simulink model "sampleModel1986"  (R2022a)
settings: Solver=FixedStepAuto  StartTime=0.0  StopTime=10.0  RelTol=1e-3
undefined symbols (not defined in the file): DiscIntNeverNeededParam, magnitude, Newton, Raphson
libraries: simulink x65, slpidlib x29
(part 1 of 4)
settings Model: SimulationMode=software-in-the-loop (sil)  Creator=lenovo  LastModifiedBy=TSMC
settings DataIOCC: InspectSignalLogs=on  SignalLoggingName=logsOut
settings OptimizationCC: DefaultParameterBehavior=Inlined  EnhancedBackFolding=on  PassReuseOutputArgsAs=Individual arguments  ZeroExternalMemoryAtStartup=off  ZeroInternalMemoryAtStartup=off  OptimizeBlockOrder=speed  DifferentSizesBufferReuse=on  OptimizationCustomize=off  EfficientTunableParamExpr=on
settings DebuggingCC: ParameterTunabilityLossMsg=error  UnconnectedInputMsg=warning  UnconnectedOutputMsg=warning  UnconnectedLineMsg=warning
settings ModelReferenceCC: UpdateModelReferenceTargets=Force
settings SFSimCC: MATLABDynamicMemAlloc=off
settings RTWCC: SystemTargetFile=ert.tlc  TemplateMakefile=ert_default_tmf  GenerateReport=on  IncludeHyperlinkInReport=on  GenerateTraceInfo=on  DLArmComputeVersion=19.05
settings CodeAppCC: ForceParamTrailComments=on  IgnoreCustomStorageClasses=off  OperatorAnnotations=on  SimulinkDataObjDesc=on  SFDataObjDesc=on  InsertBlockDesc=on
settings ERTTargetCC: TargetLangStandard=C99 (ISO)  GenerateSampleERTMain=on  SupportContinuousTime=on  InlinedParameterPlacement=NonHierarchical  ERTCustomFileTemplate=example_file_process.tlc

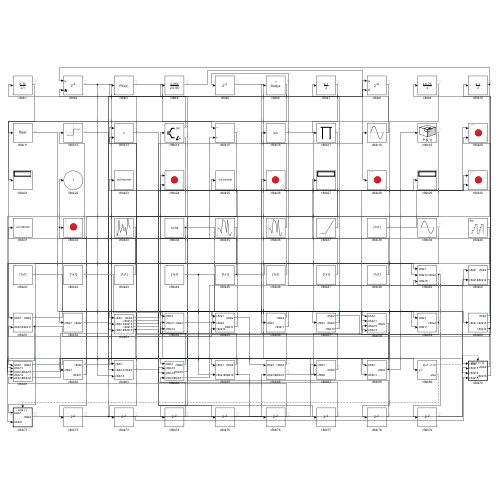
[thumbnail: Simulink's stored preview of the top-level diagram]
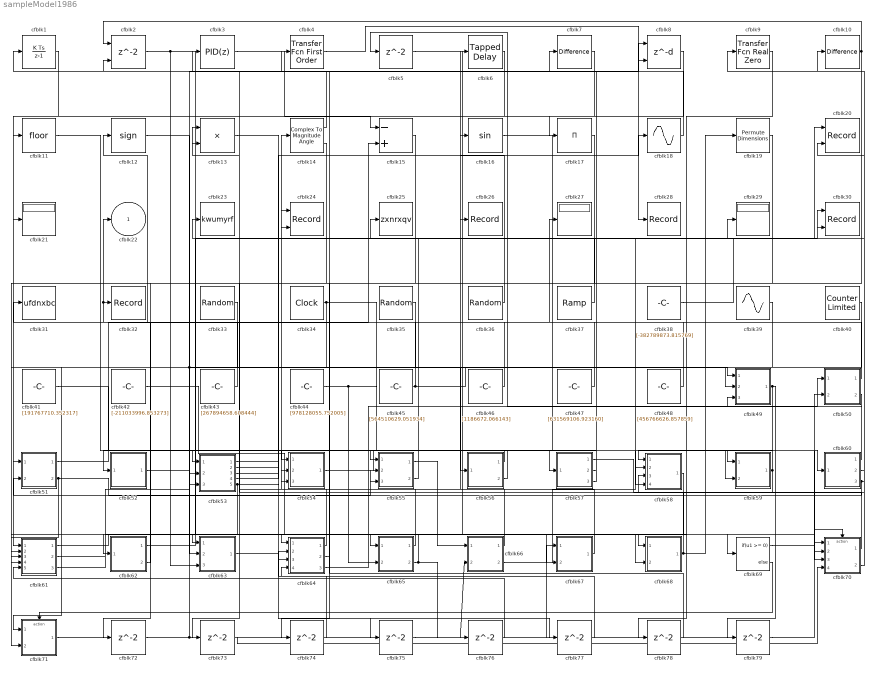
== system sampleModel1986 ==
  cfblk1 : DiscreteIntegrator  ICPrevOutput=DiscIntNeverNeededParam  ICPrevScaledInput=DiscIntNeverNeededParam
  cfblk10 : simulink/Discrete/Difference  ICPrevInput=0.0  OutMin=[]  OutMax=[]  OutDataTypeStr=Inherit: Inherit via back propagation  OutDataType=fixdt(1, 16)  OutScaling=2^-10  DoSatur=off
  cfblk11 : Rounding
  cfblk12 : Signum
  cfblk13 : Product  Inputs=**
  cfblk14 : ComplexToMagnitudeAngle
  cfblk15 : Sum  Inputs=-+
  cfblk16 : Trigonometry
  cfblk17 : Product  Inputs=*
  cfblk18 : Sin  TimeSource=Use external signal  SampleTime=0
  cfblk19 : PermuteDimensions
  cfblk2 : Delay  ShowEnablePort=on  SampleTime=1
      settings: InputPortMap=u0,e6
  cfblk20 : Record  FileSettingsInternal="{\"entries\":[{\"content\":{\"excelSettings\":{\"content\":{},\"type\":\"Streamout.ExcelSettings\"}},\"type\":\"Streamout.FileSettingStorage\",\"uuid\":\"1dca6e3d-3929-4a9b-a58f-98e31c8e366e\"}],\"packageUris\":[\"http://schema.mathworks.com/mf0/streamout_blocks/R2020a\"],\"version\":\"1.0\"}"  Layout=[1 1]  SignalsInternal="{\"entries\":[{\"content\":{\"signals\":[]},\"type\":\"RecordBlkView.InputSignals\",\"uuid\":\"f96b82a6-c829-4707-99bd-2f6ef44443c5\"}],\"packageUris\":[\"http://schema.mathworks.com/mf0/streamout_blocks/R2020a\"],\"version\":\"1.0\"}"  VisualizationBindings="{\"xyplotplugin\":{\"info\":[{\"series\":[],\"subplotID\":1}]}}"  CompatibilityTag=XY  st=-1
  cfblk21 : Display
  cfblk23 : ToWorkspace  VariableName=kwumyrf  SaveFormat=Timeseries  SampleTime=-1
  cfblk24 : Record  FileSettingsInternal="{\"entries\":[{\"content\":{\"excelSettings\":{\"content\":{},\"type\":\"Streamout.ExcelSettings\"}},\"type\":\"Streamout.FileSettingStorage\",\"uuid\":\"2952f6c9-f0ad-4b3b-947f-ff8e5daf63b8\"}],\"packageUris\":[\"http://schema.mathworks.com/mf0/streamout_blocks/R2020a\"],\"version\":\"1.0\"}"  Layout=[1 1]  SignalsInternal="{\"entries\":[{\"content\":{\"signals\":[]},\"type\":\"RecordBlkView.InputSignals\",\"uuid\":\"72db522a-7474-45f0-8336-b7d99dcf0ae2\"}],\"packageUris\":[\"http://schema.mathworks.com/mf0/streamout_blocks/R2020a\"],\"version\":\"1.0\"}"  VisualizationBindings="{\"xyplotplugin\":{\"info\":[{\"series\":[],\"subplotID\":1}]}}"  CompatibilityTag=XY  st=-1
  cfblk25 : ToWorkspace  VariableName=zxnrxqv  SaveFormat=Timeseries  SampleTime=-1
  cfblk26 : Record  FileSettingsInternal="{\"entries\":[{\"content\":{\"excelSettings\":{\"content\":{},\"type\":\"Streamout.ExcelSettings\"}},\"type\":\"Streamout.FileSettingStorage\",\"uuid\":\"125c1273-ce01-40e0-820a-1ab6df99f7c8\"}],\"packageUris\":[\"http://schema.mathworks.com/mf0/streamout_blocks/R2020a\"],\"version\":\"1.0\"}"  SignalsInternal="{\"entries\":[{\"content\":{\"signals\":[]},\"type\":\"RecordBlkView.InputSignals\",\"uuid\":\"39647610-03c1-4d8e-aa54-680a15d5938d\"}],\"packageUris\":[\"http://schema.mathworks.com/mf0/streamout_blocks/R2020a\"],\"version\":\"1.0\"}"  VisualizationBindings="{\"sparklinesplugin\":{\"info\":[{\"bindingParametersList\":[],\"subplotID\":1}]}}"
  cfblk27 : Display
  cfblk28 : Record  FileSettingsInternal="{\"entries\":[{\"content\":{\"excelSettings\":{\"content\":{},\"type\":\"Streamout.ExcelSettings\"}},\"type\":\"Streamout.FileSettingStorage\",\"uuid\":\"d5079e4d-954f-4e3f-aebb-353b75416782\"}],\"packageUris\":[\"http://schema.mathworks.com/mf0/streamout_blocks/R2020a\"],\"version\":\"1.0\"}"  SignalsInternal="{\"entries\":[{\"content\":{\"signals\":[]},\"type\":\"RecordBlkView.InputSignals\",\"uuid\":\"3476c6fd-dd80-4faf-a5c2-c4212778116c\"}],\"packageUris\":[\"http://schema.mathworks.com/mf0/streamout_blocks/R2020a\"],\"version\":\"1.0\"}"  VisualizationBindings="{\"sparklinesplugin\":{\"info\":[{\"bindingParametersList\":[],\"subplotID\":1}]}}"
  cfblk29 : Display
  cfblk3 : slpidlib/PID Controller  Controller=PID  Form=Parallel  TimeDomain=Discrete-time  UseExternalTs=off  SampleTime=1  IntegratorMethod=Forward Euler  FilterMethod=Forward Euler  ControllerParametersSource=internal  P=1  I=1  UseKiTs=off  D=0  N=100  UseFilter=on  TunerSelectOption=Transfer Function Based (PID Tuner App)  InitialConditionSource=internal  InitialConditionForIntegrator=0  InitialConditionForFilter=0  DifferentiatorICPrevScaledInput=0  ExternalReset=none  TrackingMode=off  Kt=1  LimitOutput=off  SatLimitsSource=internal  UpperSaturationLimit=inf  LowerSaturationLimit=-inf  LinearizeAsGain=off  AntiWindupMode=none  Kb=1  POutMin=[]  POutMax=[]  IOutMin=[]  IOutMax=[]  DOutMin=[]  DOutMax=[]  NOutMin=[]  NOutMax=[]  SumOutMin=[]  SumOutMax=[]  SaturationOutMin=[]  SaturationOutMax=[]  PParamMin=[]  PParamMax=[]  IParamMin=[]  IParamMax=[]  DParamMin=[]  DParamMax=[]  NParamMin=[]  NParamMax=[]  KbParamMin=[]  KbParamMax=[]  KtParamMin=[]  KtParamMax=[]  KbOutMin=[]  KbOutMax=[]  KtOutMin=[]  KtOutMax=[]  IntegratorOutMin=[]  IntegratorOutMax=[]  FilterOutMin=[]  FilterOutMax=[]  SumI1OutMin=[]  SumI1OutMax=[]  SumI2OutMin=[]  SumI2OutMax=[]  SumI3OutMin=[]  SumI3OutMax=[]  SumI4OutMin=[]  SumI4OutMax=[]  SumDOutMin=[]  SumDOutMax=[]  DifferentiatorOutMin=[]  DifferentiatorOutMax=[]  FilterDiffOutCoefMin=[]  FilterDiffOutCoefMax=[]  ReciprocalOutMin=[]  ReciprocalOutMax=[]  SumDenOutMin=[]  SumDenOutMax=[]  SumNumOutMin=[]  SumNumOutMax=[]  DivideOutMin=[]  DivideOutMax=[]  UdiffTsProdOutMin=[]  UdiffTsProdOutMax=[]  NTsProdOutMin=[]  NTsProdOutMax=[]  UintegralTsProdOutMin=[]  UintegralTsProdOutMax=[]  UngainTsProdOutMin=[]  UngainTsProdOutMax=[]  IntegratorContinuousStateAttributes=''  IntegratorStateMustResolveToSignalObject=off  IntegratorRTWStateStorageClass=Auto  FilterContinuousStateAttributes=''  FilterStateMustResolveToSignalObject=off  FilterRTWStateStorageClass=Auto  ParallelPVariant=InternalParameters  IdealPVariant=Disabled  IVariant=InternalParameters  DVariant=InternalParameters  IntegratorVariant=Discrete  SatVariant=Disabled  AWVariant=Passthrough  PCopyVariant=Disabled  TRVariant=Disabled  FdbkBlocksVariant=Forward  IdealPFdbkVariant=Disabled  SatFdbkVariant=Disabled  DerivativeFilterVariant=ForwardEulerFilter  NVariant=InternalParameters  NCopyVariant=Disabled  FilterICVariant=InternalICsFilter  IntegratorICVariant=InternalICs  ExternalResetVariant=Disabled  TRSumVariant=Passthrough  SumFdbkVariant=Disabled  SumVariant=Sum_PID  TsampFilterVariant=InternalTs  TsampNgainVariant=Passthrough  TsampIntegralVariant=Passthrough  ExternalSaturationOutDataTypeStr=Inherit: Same as second input  aMode=0
  cfblk30 : Record  FileSettingsInternal="{\"entries\":[{\"content\":{\"excelSettings\":{\"content\":{},\"type\":\"Streamout.ExcelSettings\"}},\"type\":\"Streamout.FileSettingStorage\",\"uuid\":\"e2760d90-3872-4efb-b71f-af873bcd0c0f\"}],\"packageUris\":[\"http://schema.mathworks.com/mf0/streamout_blocks/R2020a\"],\"version\":\"1.0\"}"  Layout=[1 1]  SignalsInternal="{\"entries\":[{\"content\":{\"signals\":[]},\"type\":\"RecordBlkView.InputSignals\",\"uuid\":\"4f91cc43-4657-47a6-9057-0df5bd7a9694\"}],\"packageUris\":[\"http://schema.mathworks.com/mf0/streamout_blocks/R2020a\"],\"version\":\"1.0\"}"  VisualizationBindings="{\"xyplotplugin\":{\"info\":[{\"series\":[],\"subplotID\":1}]}}"  CompatibilityTag=XY  st=-1
  cfblk31 : ToWorkspace  VariableName=ufdnxbc  SaveFormat=Timeseries  SampleTime=-1
  cfblk32 : Record  FileSettingsInternal="{\"entries\":[{\"content\":{\"excelSettings\":{\"content\":{},\"type\":\"Streamout.ExcelSettings\"}},\"type\":\"Streamout.FileSettingStorage\",\"uuid\":\"319a848f-b9c4-4916-ac33-385dec724fbf\"}],\"packageUris\":[\"http://schema.mathworks.com/mf0/streamout_blocks/R2020a\"],\"version\":\"1.0\"}"  SignalsInternal="{\"entries\":[{\"content\":{\"signals\":[]},\"type\":\"RecordBlkView.InputSignals\",\"uuid\":\"3da1b3d0-60d1-46be-bad3-5ce6aab02480\"}],\"packageUris\":[\"http://schema.mathworks.com/mf0/streamout_blocks/R2020a\"],\"version\":\"1.0\"}"  VisualizationBindings="{\"sparklinesplugin\":{\"info\":[{\"bindingParametersList\":[],\"subplotID\":1}]}}"
  cfblk33 : UniformRandomNumber  Minimum=[-1660380243.900626]  Maximum=[7164102365.047249]  Seed=[69049731.000000]  SampleTime=0.1
  cfblk34 : DigitalClock
  cfblk35 : RandomNumber  Mean=[-39556.035866]  Variance=[56886.779611]  Seed=[852067175.000000]  SampleTime=0.1
  cfblk36 : RandomNumber  Mean=[-57488.389087]  Variance=[56185.308516]  Seed=[940335256.000000]  SampleTime=0.1
  cfblk37 : simulink/Sources/Ramp  slope=[8074.641481]  start=[17.613645]  InitialOutput=[-350516.986257]
  cfblk38 : Constant  Value=[-382789873.815769]  SampleTime=1
  cfblk39 : Sin  Amplitude=[560591672.625923]  Bias=[-94874390.999346]  SampleTime=0
  cfblk4 : simulink/Discrete/Transfer Fcn First Order  PoleZ=0.95  ICPrevOutput=0.0  DoSatur=off
  cfblk40 : simulink/Sources/Counter Limited  uplimit=[971.000000]  tsamp=-1
  cfblk41 : Constant  Value=[191767710.352317]  SampleTime=1
  cfblk42 : Constant  Value=[-211033996.853273]  SampleTime=1
  cfblk43 : Constant  Value=[267894658.608444]  SampleTime=1
  cfblk44 : Constant  Value=[978128055.752005]  SampleTime=1
  cfblk45 : Constant  Value=[564510629.051934]  SampleTime=1
  cfblk46 : Constant  Value=[1186672.066143]  SampleTime=1
  cfblk47 : Constant  Value=[631569106.923160]  SampleTime=1
  cfblk48 : Constant  Value=[456766626.857859]  SampleTime=1
  cfblk49 : Subsystem
  cfblk{5,72..79} (9 alike) : Delay  SampleTime=1
  cfblk50 : Subsystem
  cfblk51 : Subsystem
  cfblk52 : Subsystem
  cfblk53 : Subsystem
  cfblk54 : Subsystem
  cfblk55 : Subsystem
  cfblk56 : Subsystem
  cfblk57 : Subsystem
  cfblk58 : Subsystem
  cfblk59 : Subsystem
  cfblk6 : simulink/Discrete/Tapped Delay  vinit=0.0  samptime=-1  NumDelays=1  DelayOrder=Oldest  includeCurrent=off
  cfblk60 : Subsystem
  cfblk61 : Subsystem
  cfblk62 : Subsystem
  cfblk63 : Subsystem
  cfblk64 : Subsystem
  cfblk65 : Subsystem
  cfblk66 : Subsystem
  cfblk67 : Subsystem
  cfblk68 : Subsystem
  cfblk69 : If  IfExpression=u1 >= 0  SampleTime=1
  cfblk7 : simulink/Discrete/Difference  ICPrevInput=0.0  OutMin=[]  OutMax=[]  OutDataTypeStr=Inherit: Inherit via back propagation  OutDataType=fixdt(1, 16)  OutScaling=2^-10  DoSatur=off
  cfblk70 : Subsystem  TreatAsAtomicUnit=on
  cfblk71 : Subsystem  TreatAsAtomicUnit=on
  cfblk8 : Delay  DelayLengthSource=Input port  SampleTime=1
      settings: InputPortMap=u0,p1
  cfblk9 : simulink/Discrete/Transfer Fcn Real Zero  ZeroZ=0.75  ICPrevInput=0.0  DoSatur=off
      settings: SourceProductBaseCode=SL
  cfblk22 : Outport
  wires:
  cfblk43/1 -> cfblk22/1, cfblk32/1
  cfblk55/1(cfblk2) -> cfblk66/1(cfblk1)
  cfblk6/1 -> cfblk61/1(cfblk1)
  cfblk59/1(cfblk2) -> cfblk58/1(cfblk1), cfblk55/3(cfblk10)
  cfblk60/1(cfblk2) -> cfblk5/1
  cfblk57/1(cfblk2) -> cfblk10/1
  cfblk16/1 -> cfblk58/2(cfblk11)
  cfblk4/1 -> cfblk28/1
  cfblk9/1 -> cfblk68/1(cfblk1)
  cfblk5/1 -> cfblk69/1
  cfblk2/1 -> cfblk64/1(cfblk1), cfblk63/3(cfblk13)
  cfblk18/1 -> cfblk7/1
  cfblk71/1(cfblk2) -> cfblk66/2(cfblk15), cfblk53/2(cfblk11)
  cfblk56/1(cfblk2) -> cfblk52/1(cfblk1)
  cfblk54/1(cfblk2) -> cfblk60/1(cfblk1)
  cfblk60/2(cfblk13) -> cfblk9/1
  cfblk44/1 -> cfblk70/1(cfblk1), cfblk65/2(cfblk15)
  cfblk68/1(cfblk2) -> cfblk13/1, cfblk19/1
  cfblk67/1(cfblk2) -> cfblk6/1
  cfblk61/1(cfblk2) -> cfblk68/2(cfblk11)
  cfblk41/1 -> cfblk57/1(cfblk1)
  cfblk65/1(cfblk2) -> cfblk13/2
  cfblk40/1 -> cfblk56/1(cfblk1)
  cfblk42/1 -> cfblk70/3(cfblk14)
  cfblk8/1 -> cfblk17/1
  cfblk62/1(cfblk2) -> cfblk30/1
  cfblk33/1 -> cfblk71/1(cfblk1), cfblk53/3(cfblk12)
  cfblk3/1 -> cfblk15/1
  cfblk14/1 -> cfblk1/1
  cfblk1/1 -> cfblk21/1
  cfblk60/3(cfblk14) -> cfblk25/1, cfblk51/2(cfblk10)
  cfblk62/2(cfblk11) -> cfblk31/1
  cfblk7/1 -> cfblk11/1
  cfblk45/1 -> cfblk49/1(cfblk1), cfblk3/1
  cfblk61/2(cfblk15) -> cfblk65/1(cfblk1)
  cfblk35/1 -> cfblk64/3(cfblk14)
  cfblk12/1 -> cfblk49/2(cfblk14)
  cfblk56/2(cfblk11) -> cfblk53/1(cfblk1)
  cfblk39/1 -> cfblk61/2(cfblk11)
  cfblk50/1(cfblk2) -> cfblk27/1
  cfblk38/1 -> cfblk20/1
  cfblk10/1 -> cfblk2/1, cfblk62/1(cfblk1)
  cfblk70/1(cfblk2) -> cfblk58/3(cfblk12)
  cfblk66/1(cfblk2) -> cfblk14/1
  cfblk49/1(cfblk2) -> cfblk78/1, cfblk79/1
  cfblk46/1 -> cfblk24/1
  cfblk50/2(cfblk14) -> cfblk49/3(cfblk15)
  cfblk15/1 -> cfblk71/2(cfblk8)
  cfblk47/1 -> cfblk12/1
  cfblk36/1 -> cfblk16/1
  cfblk57/2(cfblk9) -> cfblk54/1(cfblk1)
  cfblk65/2(cfblk16) -> cfblk63/1(cfblk1), cfblk76/1
  cfblk70/2(cfblk16) -> cfblk20/2
  cfblk13/1 -> cfblk55/1(cfblk1)
  cfblk66/2(cfblk16) -> cfblk30/2
  cfblk48/1 -> cfblk26/1
  cfblk17/1 -> cfblk63/2(cfblk12)
  cfblk64/1(cfblk2) -> cfblk54/2(cfblk11)
  cfblk57/3(cfblk10) -> cfblk4/1
  cfblk61/3(cfblk16) -> cfblk8/1
  cfblk52/1(cfblk2) -> cfblk8/2
  cfblk64/2(cfblk16) -> cfblk54/3(cfblk12)
  cfblk11/1 -> cfblk58/4(cfblk13)
  cfblk53/1(cfblk2) -> cfblk59/1(cfblk1)
  cfblk51/1(cfblk2) -> cfblk15/2
  cfblk37/1 -> cfblk23/1
  cfblk64/3(cfblk17) -> cfblk50/1(cfblk1)
  cfblk51/2(cfblk11) -> cfblk61/3(cfblk12), cfblk55/2(cfblk9)
  cfblk53/2(cfblk13) -> cfblk67/2(cfblk8)
  cfblk53/3(cfblk14) -> cfblk18/1
  cfblk34/1 -> cfblk51/1(cfblk1), cfblk59/2(cfblk11)
  cfblk55/2(cfblk11) -> cfblk24/2
  cfblk53/4(cfblk15) -> cfblk29/1
  cfblk53/5(cfblk16) -> cfblk61/4(cfblk13), cfblk77/1
  cfblk69/1 -> cfblk70/Action
  cfblk69/2 -> cfblk71/Action
  cfblk58/1(cfblk2) -> cfblk72/1
  cfblk72/1 -> cfblk70/2(cfblk13)
  cfblk14/2 -> cfblk73/1
  cfblk73/1 -> cfblk70/4(cfblk15)
  cfblk19/1 -> cfblk74/1
  cfblk74/1 -> cfblk64/2(cfblk13)
  cfblk63/1(cfblk2) -> cfblk75/1
  cfblk75/1 -> cfblk67/1(cfblk1)
  cfblk76/1 -> cfblk61/5(cfblk14)
  cfblk77/1 -> cfblk64/4(cfblk15)
  cfblk78/1 -> cfblk2/2
  cfblk79/1 -> cfblk50/2(cfblk13)

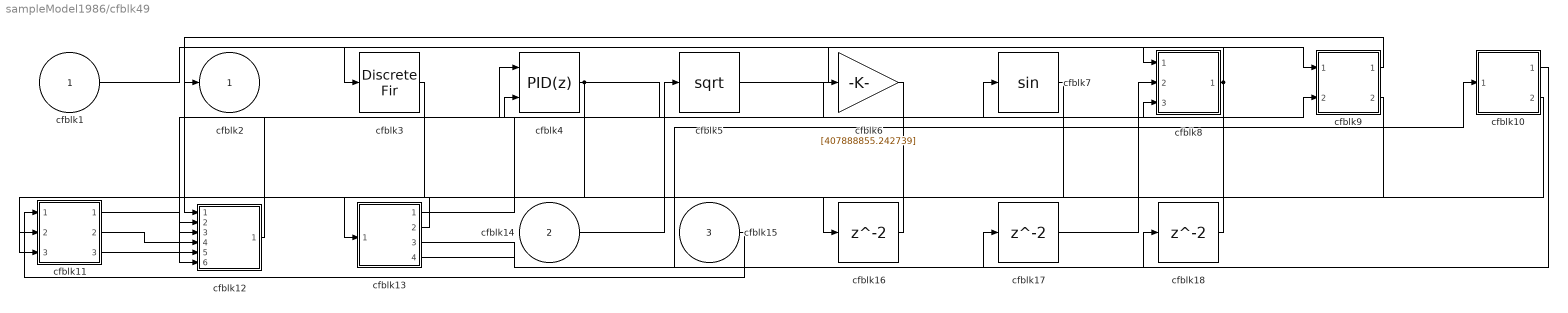
== system sampleModel1986/cfblk49 ==
  cfblk1 : Inport
  cfblk14 : Inport  Port=2
  cfblk15 : Inport  Port=3
  cfblk10 : Subsystem
  cfblk11 : Subsystem
  cfblk12 : Subsystem
  cfblk13 : Subsystem
  cfblk16 : Delay  SampleTime=1
  cfblk17 : Delay  SampleTime=1
  cfblk18 : Delay  SampleTime=1
  cfblk3 : DiscreteFir  SampleTime=1
  cfblk4 : slpidlib/PID Controller (2DOF)  Controller=PID  Form=Parallel  TimeDomain=Discrete-time  UseExternalTs=off  SampleTime=1  IntegratorMethod=Forward Euler  FilterMethod=Forward Euler  ControllerParametersSource=internal  P=1  I=1  UseKiTs=off  D=0  N=100  UseFilter=on  b=1  c=1  TunerSelectOption=Transfer Function Based (PID Tuner App)  InitialConditionSource=internal  InitialConditionForIntegrator=0  InitialConditionForFilter=0  DifferentiatorICPrevScaledInput=0  ExternalReset=none  TrackingMode=off  Kt=1  LimitOutput=off  SatLimitsSource=internal  UpperSaturationLimit=inf  LowerSaturationLimit=-inf  LinearizeAsGain=off  AntiWindupMode=none  Kb=1  POutMin=[]  POutMax=[]  IOutMin=[]  IOutMax=[]  DOutMin=[]  DOutMax=[]  NOutMin=[]  NOutMax=[]  bOutMin=[]  bOutMax=[]  cOutMin=[]  cOutMax=[]  SumOutMin=[]  SumOutMax=[]  SaturationOutMin=[]  SaturationOutMax=[]  PParamMin=[]  PParamMax=[]  IParamMin=[]  IParamMax=[]  DParamMin=[]  DParamMax=[]  NParamMin=[]  NParamMax=[]  bParamMin=[]  bParamMax=[]  cParamMin=[]  cParamMax=[]  KbParamMin=[]  KbParamMax=[]  KtParamMin=[]  KtParamMax=[]  KbOutMin=[]  KbOutMax=[]  KtOutMin=[]  KtOutMax=[]  IntegratorOutMin=[]  IntegratorOutMax=[]  FilterOutMin=[]  FilterOutMax=[]  SumI1OutMin=[]  SumI1OutMax=[]  SumI2OutMin=[]  SumI2OutMax=[]  SumI3OutMin=[]  SumI3OutMax=[]  SumI4OutMin=[]  SumI4OutMax=[]  SumDOutMin=[]  SumDOutMax=[]  Sum1OutMin=[]  Sum1OutMax=[]  Sum2OutMin=[]  Sum2OutMax=[]  Sum3OutMin=[]  Sum3OutMax=[]  DifferentiatorOutMin=[]  DifferentiatorOutMax=[]  FilterDiffOutCoefMin=[]  FilterDiffOutCoefMax=[]  ReciprocalOutMin=[]  ReciprocalOutMax=[]  SumDenOutMin=[]  SumDenOutMax=[]  SumNumOutMin=[]  SumNumOutMax=[]  DivideOutMin=[]  DivideOutMax=[]  UdiffTsProdOutMin=[]  UdiffTsProdOutMax=[]  NTsProdOutMin=[]  NTsProdOutMax=[]  UintegralTsProdOutMin=[]  UintegralTsProdOutMax=[]  UngainTsProdOutMin=[]  UngainTsProdOutMax=[]  IntegratorContinuousStateAttributes=''  IntegratorStateMustResolveToSignalObject=off  IntegratorRTWStateStorageClass=Auto  FilterContinuousStateAttributes=''  FilterStateMustResolveToSignalObject=off  FilterRTWStateStorageClass=Auto  ParallelPVariant=InternalParameters  IdealPVariant=Disabled  IVariant=InternalParameters  DVariant=InternalParameters  bVariant=InternalParameters  cVariant=InternalParameters  IntegratorVariant=Discrete  SatVariant=Disabled  AWVariant=Passthrough  PCopyVariant=Disabled  TRVariant=Disabled  FdbkBlocksVariant=Forward  IdealPFdbkVariant=Disabled  SatFdbkVariant=Disabled  DerivativeFilterVariant=ForwardEulerFilter  NVariant=InternalParameters  NCopyVariant=Disabled  FilterICVariant=InternalICsFilter  IntegratorICVariant=InternalICs  ExternalResetVariant=Disabled  TRSumVariant=Passthrough  SumFdbkVariant=Disabled  SumVariant=Sum_PID  TsampFilterVariant=InternalTs  TsampNgainVariant=Passthrough  TsampIntegralVariant=Passthrough  ExternalSaturationOutDataTypeStr=Inherit: Same as second input
      settings: SourceProductBaseCode=SL
  cfblk5 : Sqrt
  cfblk6 : Gain  Gain=[407888855.242739]
  cfblk7 : Trigonometry
  cfblk8 : Subsystem
  cfblk9 : Subsystem
  cfblk2 : Outport
  wires:
  cfblk3/1 -> cfblk13/1(cfblk1)
  cfblk5/1 -> cfblk9/1(cfblk1)
  cfblk9/1(cfblk2) -> cfblk12/1(cfblk1)
  cfblk8/1(cfblk2) -> cfblk3/1, cfblk12/6(cfblk14)
  cfblk12/1(cfblk2) -> cfblk2/1
  cfblk15/1 -> cfblk11/1(cfblk1)
  cfblk14/1 -> cfblk5/1
  cfblk13/1(cfblk2) -> cfblk6/1
  cfblk1/1 -> cfblk8/1(cfblk1)
  cfblk6/1 -> cfblk4/2
  cfblk11/1(cfblk2) -> cfblk7/1
  cfblk4/1 -> cfblk9/2(cfblk7), cfblk11/3(cfblk11)
  cfblk13/2(cfblk12) -> cfblk11/2(cfblk10)
  cfblk13/3(cfblk13) -> cfblk10/1(cfblk1)
  cfblk7/1 -> cfblk12/2(cfblk10)
  cfblk10/2(cfblk7) -> cfblk12/3(cfblk11)
  cfblk11/2(cfblk12) -> cfblk12/4(cfblk12)
  cfblk11/3(cfblk13) -> cfblk12/5(cfblk13)
  cfblk9/2(cfblk8) -> cfblk16/1
  cfblk16/1 -> cfblk4/1
  cfblk10/1(cfblk2) -> cfblk17/1
  cfblk17/1 -> cfblk8/2(cfblk11)
  cfblk13/4(cfblk14) -> cfblk18/1
  cfblk18/1 -> cfblk8/3(cfblk12)

== system sampleModel1986/cfblk50 ==
  cfblk1 : Inport
  cfblk13 : Inport  Port=2
  cfblk10 : Constant  Value=[849540447.237942]  SampleTime=1
  cfblk11 : Constant  Value=[-641366337.770098]  SampleTime=1
  cfblk12 : Subsystem
  cfblk15 : Delay  SampleTime=1
  cfblk3 : slpidlib/PID Controller (2DOF)  Controller=PID  Form=Parallel  TimeDomain=Discrete-time  UseExternalTs=off  SampleTime=1  IntegratorMethod=Forward Euler  FilterMethod=Forward Euler  ControllerParametersSource=internal  P=1  I=1  UseKiTs=off  D=0  N=100  UseFilter=on  b=1  c=1  TunerSelectOption=Transfer Function Based (PID Tuner App)  InitialConditionSource=internal  InitialConditionForIntegrator=0  InitialConditionForFilter=0  DifferentiatorICPrevScaledInput=0  ExternalReset=none  TrackingMode=off  Kt=1  LimitOutput=off  SatLimitsSource=internal  UpperSaturationLimit=inf  LowerSaturationLimit=-inf  LinearizeAsGain=off  AntiWindupMode=none  Kb=1  POutMin=[]  POutMax=[]  IOutMin=[]  IOutMax=[]  DOutMin=[]  DOutMax=[]  NOutMin=[]  NOutMax=[]  bOutMin=[]  bOutMax=[]  cOutMin=[]  cOutMax=[]  SumOutMin=[]  SumOutMax=[]  SaturationOutMin=[]  SaturationOutMax=[]  PParamMin=[]  PParamMax=[]  IParamMin=[]  IParamMax=[]  DParamMin=[]  DParamMax=[]  NParamMin=[]  NParamMax=[]  bParamMin=[]  bParamMax=[]  cParamMin=[]  cParamMax=[]  KbParamMin=[]  KbParamMax=[]  KtParamMin=[]  KtParamMax=[]  KbOutMin=[]  KbOutMax=[]  KtOutMin=[]  KtOutMax=[]  IntegratorOutMin=[]  IntegratorOutMax=[]  FilterOutMin=[]  FilterOutMax=[]  SumI1OutMin=[]  SumI1OutMax=[]  SumI2OutMin=[]  SumI2OutMax=[]  SumI3OutMin=[]  SumI3OutMax=[]  SumI4OutMin=[]  SumI4OutMax=[]  SumDOutMin=[]  SumDOutMax=[]  Sum1OutMin=[]  Sum1OutMax=[]  Sum2OutMin=[]  Sum2OutMax=[]  Sum3OutMin=[]  Sum3OutMax=[]  DifferentiatorOutMin=[]  DifferentiatorOutMax=[]  FilterDiffOutCoefMin=[]  FilterDiffOutCoefMax=[]  ReciprocalOutMin=[]  ReciprocalOutMax=[]  SumDenOutMin=[]  SumDenOutMax=[]  SumNumOutMin=[]  SumNumOutMax=[]  DivideOutMin=[]  DivideOutMax=[]  UdiffTsProdOutMin=[]  UdiffTsProdOutMax=[]  NTsProdOutMin=[]  NTsProdOutMax=[]  UintegralTsProdOutMin=[]  UintegralTsProdOutMax=[]  UngainTsProdOutMin=[]  UngainTsProdOutMax=[]  IntegratorContinuousStateAttributes=''  IntegratorStateMustResolveToSignalObject=off  IntegratorRTWStateStorageClass=Auto  FilterContinuousStateAttributes=''  FilterStateMustResolveToSignalObject=off  FilterRTWStateStorageClass=Auto  ParallelPVariant=InternalParameters  IdealPVariant=Disabled  IVariant=InternalParameters  DVariant=InternalParameters  bVariant=InternalParameters  cVariant=InternalParameters  IntegratorVariant=Discrete  SatVariant=Disabled  AWVariant=Passthrough  PCopyVariant=Disabled  TRVariant=Disabled  FdbkBlocksVariant=Forward  IdealPFdbkVariant=Disabled  SatFdbkVariant=Disabled  DerivativeFilterVariant=ForwardEulerFilter  NVariant=InternalParameters  NCopyVariant=Disabled  FilterICVariant=InternalICsFilter  IntegratorICVariant=InternalICs  ExternalResetVariant=Disabled  TRSumVariant=Passthrough  SumFdbkVariant=Disabled  SumVariant=Sum_PID  TsampFilterVariant=InternalTs  TsampNgainVariant=Passthrough  TsampIntegralVariant=Passthrough  ExternalSaturationOutDataTypeStr=Inherit: Same as second input
      settings: SourceProductBaseCode=SL
  cfblk4 : Delay  ShowEnablePort=on  SampleTime=1
      settings: InputPortMap=u0,e6
  cfblk5 : simulink/Discrete/Transfer Fcn Lead or Lag  PoleZ=0.95  ZeroZ=0.75  ICPrevOutput=0.0  ICPrevInput=0.0  DoSatur=off
      settings: SourceProductBaseCode=SL
  cfblk6 : Reshape
  cfblk7 : Assignment  DiagnosticForDimensions=Warning  IndexOptions=Index vector (dialog)  Indices=1  OutputSizes=1
  cfblk8 : Sqrt  Operator=rSqrt  AlgorithmType=Newton-Raphson
  cfblk9 : Abs  SaturateOnIntegerOverflow=off
  cfblk2 : Outport
  cfblk14 : Outport  Port=2
  wires:
  cfblk5/1 -> cfblk7/1
  cfblk4/1 -> cfblk8/1
  cfblk13/1 -> cfblk4/1
  cfblk6/1 -> cfblk12/1(cfblk1)
  cfblk11/1 -> cfblk2/1
  cfblk8/1 -> cfblk5/1
  cfblk9/1 -> cfblk3/1
  cfblk12/2(cfblk9) -> cfblk3/2
  cfblk7/1 -> cfblk9/1
  cfblk10/1 -> cfblk4/2
  cfblk3/1 -> cfblk14/1
  cfblk1/1 -> cfblk7/2
  cfblk12/1(cfblk2) -> cfblk15/1
  cfblk15/1 -> cfblk6/1

== system sampleModel1986/cfblk51 ==
  cfblk1 : Inport
  cfblk10 : Inport  Port=2
  cfblk12 : Delay  SampleTime=1
  cfblk13 : Delay  SampleTime=1
  cfblk14 : Delay  SampleTime=1
  cfblk3 : Math  Operator=pow
  cfblk4 : Polyval  Coefs=[ +2.081618890e-019, -1.441693666e-014, +4.719686976e-010, -8.536869453e-006, +1.621573104e-001, -8.087801117e+001 ]
  cfblk5 : Sqrt  Operator=rSqrt  AlgorithmType=Newton-Raphson
  cfblk6 : Constant  Value=[-34064911.828478]  SampleTime=1
  cfblk7 : Subsystem
  cfblk8 : Subsystem
  cfblk9 : Subsystem
  cfblk2 : Outport
  cfblk11 : Outport  Port=2
  wires:
  cfblk9/1(cfblk2) -> cfblk7/1(cfblk1)
  cfblk10/1 -> cfblk5/1
  cfblk5/1 -> cfblk4/1
  cfblk3/1 -> cfblk11/1
  cfblk6/1 -> cfblk3/1
  cfblk7/1(cfblk2) -> cfblk2/1
  cfblk4/1 -> cfblk8/1(cfblk1)
  cfblk7/2(cfblk12) -> cfblk3/2
  cfblk7/3(cfblk13) -> cfblk8/2(cfblk8)
  cfblk7/4(cfblk14) -> cfblk8/3(cfblk9)
  cfblk1/1 -> cfblk9/3(cfblk11)
  cfblk8/1(cfblk2) -> cfblk12/1
  cfblk12/1 -> cfblk9/1(cfblk1)
  cfblk8/2(cfblk10) -> cfblk13/1
  cfblk13/1 -> cfblk9/2(cfblk10)
  cfblk7/5(cfblk15) -> cfblk14/1
  cfblk14/1 -> cfblk9/4(cfblk12)

== system sampleModel1986/cfblk52 ==
  cfblk1 : Inport
  cfblk10 : Constant  Value=[650099455.593839]  SampleTime=1
  cfblk11 : Subsystem
  cfblk12 : Subsystem
  cfblk13 : Delay  SampleTime=1
  cfblk14 : Delay  SampleTime=1
  cfblk3 : DiscreteStateSpace
  cfblk4 : simulink/Discrete/Transfer Fcn First Order  PoleZ=0.95  ICPrevOutput=0.0  DoSatur=off
  cfblk5 : Gain  Gain=[-531846681.099334]
  cfblk6 : MinMax  Function=max
  cfblk7 : UnaryMinus
  cfblk8 : Sum  Inputs=-+
  cfblk9 : Constant  Value=[914222812.365636]  SampleTime=1
  cfblk2 : Outport
  wires:
  cfblk7/1 -> cfblk13/1, cfblk14/1
  cfblk5/1 -> cfblk6/1, cfblk12/2(cfblk8)
  cfblk11/1(cfblk2) -> cfblk3/1
  cfblk8/1 -> cfblk7/1
  cfblk10/1 -> cfblk2/1
  cfblk1/1 -> cfblk11/2(cfblk8)
  cfblk4/1 -> cfblk8/1
  cfblk6/1 -> cfblk11/3(cfblk9)
  cfblk3/1 -> cfblk12/1(cfblk1)
  cfblk9/1 -> cfblk5/1, cfblk8/2
  cfblk12/1(cfblk2) -> cfblk4/1
  cfblk13/1 -> cfblk11/1(cfblk1)
  cfblk14/1 -> cfblk11/4(cfblk10)

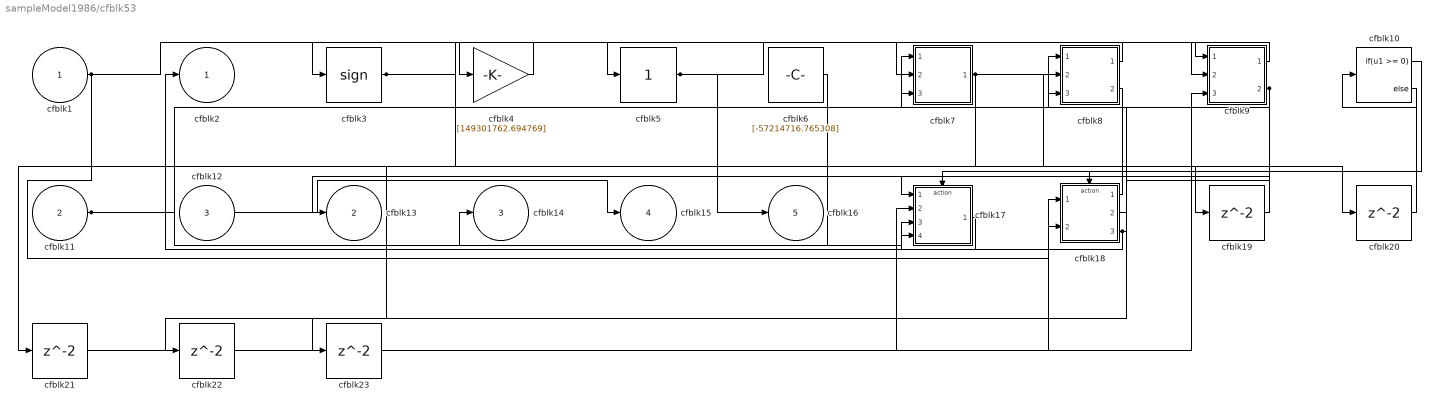
== system sampleModel1986/cfblk53 ==
  cfblk1 : Inport
  cfblk11 : Inport  Port=2
  cfblk12 : Inport  Port=3
  cfblk10 : If  IfExpression=u1 >= 0  SampleTime=1
  cfblk17 : Subsystem  TreatAsAtomicUnit=on
  cfblk18 : Subsystem  TreatAsAtomicUnit=on
  cfblk{19..23} (5 alike) : Delay  SampleTime=1
  cfblk3 : Signum
  cfblk4 : Gain  Gain=[149301762.694769]
  cfblk5 : simulink/Math Operations/Slider Gain  gain=1  low=0  high=2
  cfblk6 : Constant  Value=[-57214716.765308]  SampleTime=1
  cfblk7 : Subsystem
  cfblk8 : Subsystem
  cfblk9 : Subsystem
  cfblk2 : Outport
  cfblk13 : Outport  Port=2
  cfblk14 : Outport  Port=3
  cfblk15 : Outport  Port=4
  cfblk16 : Outport  Port=5
  wires:
  cfblk9/1(cfblk2) -> cfblk5/1
  cfblk5/1 -> cfblk16/1, cfblk7/2(cfblk13)
  cfblk4/1 -> cfblk3/1
  cfblk7/1(cfblk2) -> cfblk20/1, cfblk21/1
  cfblk17/1(cfblk2) -> cfblk2/1
  cfblk18/1(cfblk2) -> cfblk8/1(cfblk1)
  cfblk6/1 -> cfblk14/1
  cfblk12/1 -> cfblk15/1
  cfblk3/1 -> cfblk9/2(cfblk6), cfblk7/3(cfblk14), cfblk19/1
  cfblk11/1 -> cfblk8/3(cfblk8), cfblk17/3(cfblk11)
  cfblk8/1(cfblk2) -> cfblk4/1
  cfblk9/2(cfblk8) -> cfblk13/1, cfblk22/1
  cfblk1/1 -> cfblk18/1(cfblk1), cfblk9/1(cfblk1)
  cfblk18/2(cfblk11) -> cfblk17/1(cfblk1)
  cfblk18/3(cfblk12) -> cfblk7/1(cfblk1), cfblk17/4(cfblk12)
  cfblk10/1 -> cfblk17/Action
  cfblk10/2 -> cfblk18/Action
  cfblk19/1 -> cfblk8/2(cfblk7)
  cfblk20/1 -> cfblk10/1
  cfblk21/1 -> cfblk9/3(cfblk7)
  cfblk22/1 -> cfblk17/2(cfblk10)
  cfblk8/2(cfblk9) -> cfblk23/1
  cfblk23/1 -> cfblk18/2(cfblk10)

== system sampleModel1986/cfblk54 ==
  cfblk1 : Inport
  cfblk11 : Inport  Port=2
  cfblk12 : Inport  Port=3
  cfblk10 : Subsystem
  cfblk13 : Delay  SampleTime=1
  cfblk3 : simulink/Discrete/Tapped Delay  vinit=0.0  samptime=-1  NumDelays=1  DelayOrder=Oldest  includeCurrent=off
  cfblk4 : simulink/Discrete/Transfer Fcn First Order  PoleZ=0.95  ICPrevOutput=0.0  DoSatur=off
  cfblk5 : DiscreteZeroPole  Poles=[0 0.5]  Gain=1
  cfblk6 : simulink/Discrete/Tapped Delay  vinit=0.0  samptime=-1  NumDelays=1  DelayOrder=Oldest  includeCurrent=off
  cfblk7 : simulink/Math Operations/MinMax Running Resettable  Function=min  vinit=0.0
  cfblk8 : simulink/Math Operations/Slider Gain  gain=1  low=0  high=2
  cfblk9 : UnaryMinus
  cfblk2 : Outport
  wires:
  cfblk9/1 -> cfblk6/1
  cfblk4/1 -> cfblk2/1
  cfblk3/1 -> cfblk10/1(cfblk1)
  cfblk8/1 -> cfblk9/1
  cfblk12/1 -> cfblk8/1
  cfblk11/1 -> cfblk3/1
  cfblk10/1(cfblk2) -> cfblk5/1
  cfblk5/1 -> cfblk7/1
  cfblk7/1 -> cfblk4/1, cfblk13/1
  cfblk6/1 -> cfblk7/2
  cfblk1/1 -> cfblk10/2(cfblk9)
  cfblk13/1 -> cfblk10/3(cfblk10)

== system sampleModel1986/cfblk55 ==
  cfblk1 : Inport
  cfblk9 : Inport  Port=2
  cfblk10 : Inport  Port=3
  cfblk3 : Delay  DelayLengthSource=Input port  SampleTime=1
      settings: InputPortMap=u0,p1
  cfblk4 : Polyval  Coefs=[ +2.081618890e-019, -1.441693666e-014, +4.719686976e-010, -8.536869453e-006, +1.621573104e-001, -8.087801117e+001 ]
  cfblk5 : Math  Operator=log10
  cfblk6 : Constant  Value=[495403200.105896]  SampleTime=1
  cfblk7 : Constant  Value=[700007903.664398]  SampleTime=1
  cfblk8 : Subsystem
  cfblk2 : Outport
  cfblk11 : Outport  Port=2
  wires:
  cfblk6/1 -> cfblk3/1
  cfblk1/1 -> cfblk5/1
  cfblk5/1 -> cfblk8/1(cfblk1)
  cfblk8/1(cfblk2) -> cfblk11/1
  cfblk9/1 -> cfblk4/1
  cfblk3/1 -> cfblk2/1
  cfblk4/1 -> cfblk8/2(cfblk13)
  cfblk7/1 -> cfblk3/2
  cfblk10/1 -> cfblk8/3(cfblk14)

== system sampleModel1986/cfblk56 ==
  cfblk1 : Inport
  cfblk10 : Subsystem
  cfblk12 : Delay  SampleTime=1
  cfblk13 : Delay  SampleTime=1
  cfblk14 : DataTypeConversion  SaturateOnIntegerOverflow=off  RndMeth=Floor
  cfblk15 : DataTypeConversion  SaturateOnIntegerOverflow=off  RndMeth=Floor
  cfblk3 : slpidlib/PID Controller  Controller=PID  Form=Parallel  TimeDomain=Discrete-time  UseExternalTs=off  SampleTime=1  IntegratorMethod=Forward Euler  FilterMethod=Forward Euler  ControllerParametersSource=internal  P=1  I=1  UseKiTs=off  D=0  N=100  UseFilter=on  TunerSelectOption=Transfer Function Based (PID Tuner App)  InitialConditionSource=internal  InitialConditionForIntegrator=0  InitialConditionForFilter=0  DifferentiatorICPrevScaledInput=0  ExternalReset=none  TrackingMode=off  Kt=1  LimitOutput=off  SatLimitsSource=internal  UpperSaturationLimit=inf  LowerSaturationLimit=-inf  LinearizeAsGain=off  AntiWindupMode=none  Kb=1  POutMin=[]  POutMax=[]  IOutMin=[]  IOutMax=[]  DOutMin=[]  DOutMax=[]  NOutMin=[]  NOutMax=[]  SumOutMin=[]  SumOutMax=[]  SaturationOutMin=[]  SaturationOutMax=[]  PParamMin=[]  PParamMax=[]  IParamMin=[]  IParamMax=[]  DParamMin=[]  DParamMax=[]  NParamMin=[]  NParamMax=[]  KbParamMin=[]  KbParamMax=[]  KtParamMin=[]  KtParamMax=[]  KbOutMin=[]  KbOutMax=[]  KtOutMin=[]  KtOutMax=[]  IntegratorOutMin=[]  IntegratorOutMax=[]  FilterOutMin=[]  FilterOutMax=[]  SumI1OutMin=[]  SumI1OutMax=[]  SumI2OutMin=[]  SumI2OutMax=[]  SumI3OutMin=[]  SumI3OutMax=[]  SumI4OutMin=[]  SumI4OutMax=[]  SumDOutMin=[]  SumDOutMax=[]  DifferentiatorOutMin=[]  DifferentiatorOutMax=[]  FilterDiffOutCoefMin=[]  FilterDiffOutCoefMax=[]  ReciprocalOutMin=[]  ReciprocalOutMax=[]  SumDenOutMin=[]  SumDenOutMax=[]  SumNumOutMin=[]  SumNumOutMax=[]  DivideOutMin=[]  DivideOutMax=[]  UdiffTsProdOutMin=[]  UdiffTsProdOutMax=[]  NTsProdOutMin=[]  NTsProdOutMax=[]  UintegralTsProdOutMin=[]  UintegralTsProdOutMax=[]  UngainTsProdOutMin=[]  UngainTsProdOutMax=[]  IntegratorContinuousStateAttributes=''  IntegratorStateMustResolveToSignalObject=off  IntegratorRTWStateStorageClass=Auto  FilterContinuousStateAttributes=''  FilterStateMustResolveToSignalObject=off  FilterRTWStateStorageClass=Auto  ParallelPVariant=InternalParameters  IdealPVariant=Disabled  IVariant=InternalParameters  DVariant=InternalParameters  IntegratorVariant=Discrete  SatVariant=Disabled  AWVariant=Passthrough  PCopyVariant=Disabled  TRVariant=Disabled  FdbkBlocksVariant=Forward  IdealPFdbkVariant=Disabled  SatFdbkVariant=Disabled  DerivativeFilterVariant=ForwardEulerFilter  NVariant=InternalParameters  NCopyVariant=Disabled  FilterICVariant=InternalICsFilter  IntegratorICVariant=InternalICs  ExternalResetVariant=Disabled  TRSumVariant=Passthrough  SumFdbkVariant=Disabled  SumVariant=Sum_PID  TsampFilterVariant=InternalTs  TsampNgainVariant=Passthrough  TsampIntegralVariant=Passthrough  ExternalSaturationOutDataTypeStr=Inherit: Same as second input  aMode=0
  cfblk4 : Gain  Gain=[366904369.123828]
  cfblk5 : Abs  SaturateOnIntegerOverflow=off
  cfblk6 : Subsystem
  cfblk7 : Subsystem
  cfblk8 : Subsystem
  cfblk9 : Subsystem
  cfblk2 : Outport
  cfblk11 : Outport  Port=2
  wires:
  cfblk7/1(cfblk2) -> cfblk8/1(cfblk1)
  cfblk1/1 -> cfblk10/1(cfblk1), cfblk6/3(cfblk15), cfblk7/2(cfblk5)
  cfblk6/1(cfblk2) -> cfblk4/1
  cfblk8/2(cfblk10) -> cfblk6/1(cfblk1)
  cfblk10/1(cfblk2) -> cfblk11/1
  cfblk10/2(cfblk12) -> cfblk9/2(cfblk15), cfblk6/5(cfblk17)
  cfblk4/1 -> cfblk5/1
  cfblk7/2(cfblk6) -> cfblk8/3(cfblk9)
  cfblk5/1 -> cfblk2/1
  cfblk9/1(cfblk2) -> cfblk6/2(cfblk14)
  cfblk9/2(cfblk17) -> cfblk7/1(cfblk1), cfblk6/4(cfblk16)
  cfblk8/1(cfblk2) -> cfblk12/1
  cfblk12/1 -> cfblk9/1(cfblk1)
  cfblk7/3(cfblk7) -> cfblk13/1
  cfblk13/1 -> cfblk9/3(cfblk16)
  cfblk3/1 -> cfblk14/1
  cfblk14/1 -> cfblk8/2(cfblk8)
  cfblk7/4(cfblk8) -> cfblk15/1
  cfblk15/1 -> cfblk3/1

== system sampleModel1986/cfblk57 ==
  cfblk1 : Inport
  cfblk{11..14} (4 alike) : Delay  SampleTime=1
  cfblk3 : DiscreteFilter  SampleTime=1
  cfblk4 : Sin  TimeSource=Use external signal  SampleTime=0
  cfblk5 : Subsystem
  cfblk6 : Subsystem
  cfblk7 : Subsystem
  cfblk8 : Subsystem
  cfblk2 : Outport
  cfblk9 : Outport  Port=2
  cfblk10 : Outport  Port=3
  wires:
  cfblk7/1(cfblk2) -> cfblk6/1(cfblk1)
  cfblk3/1 -> cfblk5/1(cfblk1), cfblk5/2(cfblk9), cfblk5/3(cfblk10)
  cfblk5/2(cfblk11) -> cfblk7/1(cfblk1)
  cfblk4/1 -> cfblk11/1, cfblk12/1, cfblk13/1
  cfblk1/1 -> cfblk7/2(cfblk8), cfblk7/3(cfblk9), cfblk9/1, cfblk8/4(cfblk11)
  cfblk5/3(cfblk12) -> cfblk6/3(cfblk11), cfblk8/2(cfblk9)
  cfblk6/1(cfblk2) -> cfblk8/1(cfblk1)
  cfblk8/1(cfblk2) -> cfblk4/1
  cfblk7/2(cfblk11) -> cfblk2/1, cfblk10/1
  cfblk11/1 -> cfblk6/2(cfblk10)
  cfblk12/1 -> cfblk8/3(cfblk10)
  cfblk13/1 -> cfblk7/4(cfblk10)
  cfblk5/1(cfblk2) -> cfblk14/1
  cfblk14/1 -> cfblk3/1

== system sampleModel1986/cfblk58 ==
  cfblk1 : Inport
  cfblk11 : Inport  Port=2
  cfblk12 : Inport  Port=3
  cfblk13 : Inport  Port=4
  cfblk10 : Subsystem
  cfblk14 : Delay  SampleTime=1
  cfblk15 : Delay  SampleTime=1
  cfblk3 : simulink/Discrete/Difference  ICPrevInput=0.0  OutMin=[]  OutMax=[]  OutDataTypeStr=Inherit: Inherit via back propagation  OutDataType=fixdt(1, 16)  OutScaling=2^-10  DoSatur=off
  cfblk4 : DotProduct  OutDataTypeStr=Inherit: Inherit via internal rule
  cfblk5 : Abs  SaturateOnIntegerOverflow=off
  cfblk6 : Constant  Value=[263448576.933128]  SampleTime=1
  cfblk7 : Constant  Value=[-111462374.336733]  SampleTime=1
  cfblk8 : Subsystem
  cfblk9 : Subsystem
  cfblk2 : Outport
  wires:
  cfblk12/1 -> cfblk3/1
  cfblk7/1 -> cfblk9/1(cfblk1)
  cfblk13/1 -> cfblk5/1, cfblk10/5(cfblk13)
  cfblk5/1 -> cfblk4/1
  cfblk9/1(cfblk2) -> cfblk4/2
  cfblk3/1 -> cfblk8/1(cfblk1), cfblk10/3(cfblk11), cfblk9/5(cfblk12)
  cfblk1/1 -> cfblk9/2(cfblk9)
  cfblk6/1 -> cfblk10/1(cfblk1)
  cfblk11/1 -> cfblk8/2(cfblk8), cfblk9/4(cfblk11)
  cfblk4/1 -> cfblk2/1, cfblk10/4(cfblk12)
  cfblk9/2(cfblk13) -> cfblk8/3(cfblk9)
  cfblk10/1(cfblk2) -> cfblk8/4(cfblk10)
  cfblk10/2(cfblk14) -> cfblk8/5(cfblk11)
  cfblk8/1(cfblk2) -> cfblk14/1
  cfblk14/1 -> cfblk10/2(cfblk10)
  cfblk10/3(cfblk15) -> cfblk15/1
  cfblk15/1 -> cfblk9/3(cfblk10)

== system sampleModel1986/cfblk59 ==
  cfblk1 : Inport
  cfblk11 : Inport  Port=2
  cfblk10 : Subsystem
  cfblk{12..15} (4 alike) : Delay  SampleTime=1
  cfblk3 : Delay  ShowEnablePort=on  SampleTime=1
      settings: InputPortMap=u0,e6
  cfblk4 : slpidlib/PID Controller (2DOF)  Controller=PID  Form=Parallel  TimeDomain=Discrete-time  UseExternalTs=off  SampleTime=1  IntegratorMethod=Forward Euler  FilterMethod=Forward Euler  ControllerParametersSource=internal  P=1  I=1  UseKiTs=off  D=0  N=100  UseFilter=on  b=1  c=1  TunerSelectOption=Transfer Function Based (PID Tuner App)  InitialConditionSource=internal  InitialConditionForIntegrator=0  InitialConditionForFilter=0  DifferentiatorICPrevScaledInput=0  ExternalReset=none  TrackingMode=off  Kt=1  LimitOutput=off  SatLimitsSource=internal  UpperSaturationLimit=inf  LowerSaturationLimit=-inf  LinearizeAsGain=off  AntiWindupMode=none  Kb=1  POutMin=[]  POutMax=[]  IOutMin=[]  IOutMax=[]  DOutMin=[]  DOutMax=[]  NOutMin=[]  NOutMax=[]  bOutMin=[]  bOutMax=[]  cOutMin=[]  cOutMax=[]  SumOutMin=[]  SumOutMax=[]  SaturationOutMin=[]  SaturationOutMax=[]  PParamMin=[]  PParamMax=[]  IParamMin=[]  IParamMax=[]  DParamMin=[]  DParamMax=[]  NParamMin=[]  NParamMax=[]  bParamMin=[]  bParamMax=[]  cParamMin=[]  cParamMax=[]  KbParamMin=[]  KbParamMax=[]  KtParamMin=[]  KtParamMax=[]  KbOutMin=[]  KbOutMax=[]  KtOutMin=[]  KtOutMax=[]  IntegratorOutMin=[]  IntegratorOutMax=[]  FilterOutMin=[]  FilterOutMax=[]  SumI1OutMin=[]  SumI1OutMax=[]  SumI2OutMin=[]  SumI2OutMax=[]  SumI3OutMin=[]  SumI3OutMax=[]  SumI4OutMin=[]  SumI4OutMax=[]  SumDOutMin=[]  SumDOutMax=[]  Sum1OutMin=[]  Sum1OutMax=[]  Sum2OutMin=[]  Sum2OutMax=[]  Sum3OutMin=[]  Sum3OutMax=[]  DifferentiatorOutMin=[]  DifferentiatorOutMax=[]  FilterDiffOutCoefMin=[]  FilterDiffOutCoefMax=[]  ReciprocalOutMin=[]  ReciprocalOutMax=[]  SumDenOutMin=[]  SumDenOutMax=[]  SumNumOutMin=[]  SumNumOutMax=[]  DivideOutMin=[]  DivideOutMax=[]  UdiffTsProdOutMin=[]  UdiffTsProdOutMax=[]  NTsProdOutMin=[]  NTsProdOutMax=[]  UintegralTsProdOutMin=[]  UintegralTsProdOutMax=[]  UngainTsProdOutMin=[]  UngainTsProdOutMax=[]  IntegratorContinuousStateAttributes=''  IntegratorStateMustResolveToSignalObject=off  IntegratorRTWStateStorageClass=Auto  FilterContinuousStateAttributes=''  FilterStateMustResolveToSignalObject=off  FilterRTWStateStorageClass=Auto  ParallelPVariant=InternalParameters  IdealPVariant=Disabled  IVariant=InternalParameters  DVariant=InternalParameters  bVariant=InternalParameters  cVariant=InternalParameters  IntegratorVariant=Discrete  SatVariant=Disabled  AWVariant=Passthrough  PCopyVariant=Disabled  TRVariant=Disabled  FdbkBlocksVariant=Forward  IdealPFdbkVariant=Disabled  SatFdbkVariant=Disabled  DerivativeFilterVariant=ForwardEulerFilter  NVariant=InternalParameters  NCopyVariant=Disabled  FilterICVariant=InternalICsFilter  IntegratorICVariant=InternalICs  ExternalResetVariant=Disabled  TRSumVariant=Passthrough  SumFdbkVariant=Disabled  SumVariant=Sum_PID  TsampFilterVariant=InternalTs  TsampNgainVariant=Passthrough  TsampIntegralVariant=Passthrough  ExternalSaturationOutDataTypeStr=Inherit: Same as second input
      settings: SourceProductBaseCode=SL
  cfblk5 : Reshape
  cfblk6 : MinMax
  cfblk7 : Rounding
  cfblk8 : simulink/Math Operations/Slider Gain  gain=1  low=0  high=2
  cfblk9 : Subsystem
  cfblk2 : Outport
  wires:
  cfblk8/1 -> cfblk4/1, cfblk6/1, cfblk13/1, cfblk14/1, cfblk15/1
  cfblk5/1 -> cfblk10/1(cfblk1), cfblk10/4(cfblk12)
  cfblk3/1 -> cfblk7/1
  cfblk10/1(cfblk2) -> cfblk9/1(cfblk1)
  cfblk9/1(cfblk2) -> cfblk3/1
  cfblk1/1 -> cfblk5/1
  cfblk6/1 -> cfblk2/1
  cfblk9/2(cfblk13) -> cfblk4/2
  cfblk7/1 -> cfblk8/1
  cfblk11/1 -> cfblk9/2(cfblk10), cfblk9/3(cfblk11)
  cfblk4/1 -> cfblk12/1
  cfblk12/1 -> cfblk10/2(cfblk10)
  cfblk13/1 -> cfblk10/3(cfblk11)
  cfblk14/1 -> cfblk9/4(cfblk12)
  cfblk15/1 -> cfblk3/2

== system sampleModel1986/cfblk60 ==
  cfblk1 : Inport
  cfblk10 : Constant  Value=[5443228.947851]  SampleTime=1
  cfblk11 : Subsystem
  cfblk12 : Subsystem
  cfblk3 : UnitDelay  HasFrameUpgradeWarning=on
  cfblk4 : simulink/Discrete/Transfer Fcn First Order  PoleZ=0.95  ICPrevOutput=0.0  DoSatur=off
  cfblk5 : DiscreteTransferFcn  SampleTime=1
  cfblk6 : Delay  ShowEnablePort=on  SampleTime=1
      settings: InputPortMap=u0,e6
  cfblk7 : Bias  Bias=[-22955398.698810]  SaturateOnIntegerOverflow=off
  cfblk8 : Sum  Inputs=+-
  cfblk9 : Constant  Value=[-793462366.403758]  SampleTime=1
  cfblk2 : Outport
  cfblk13 : Outport  Port=2
  cfblk14 : Outport  Port=3
  wires:
  cfblk6/1 -> cfblk5/1
  cfblk9/1 -> cfblk7/1
  cfblk1/1 -> cfblk4/1
  cfblk4/1 -> cfblk8/1, cfblk11/2(cfblk11)
  cfblk10/1 -> cfblk6/1, cfblk12/2(cfblk12)
  cfblk7/1 -> cfblk8/2
  cfblk8/1 -> cfblk6/2
  cfblk3/1 -> cfblk2/1
  cfblk11/1(cfblk2) -> cfblk13/1
  cfblk5/1 -> cfblk12/1(cfblk1)
  cfblk12/1(cfblk2) -> cfblk14/1
  cfblk12/2(cfblk13) -> cfblk3/1
  cfblk12/3(cfblk14) -> cfblk11/1(cfblk1)

== system sampleModel1986/cfblk61 ==
  cfblk1 : Inport
  cfblk11 : Inport  Port=2
  cfblk12 : Inport  Port=3
  cfblk13 : Inport  Port=4
  cfblk14 : Inport  Port=5
  cfblk10 : Constant  Value=[381329186.466179]  SampleTime=1
  cfblk3 : Delay  SampleTime=1
  cfblk4 : DiscreteFir  SampleTime=1
  cfblk5 : DiscreteTransferFcn  SampleTime=1
  cfblk6 : Trigonometry
  cfblk7 : Signum
  cfblk8 : PermuteDimensions
  cfblk9 : Constant  Value=[-998252840.048321]  SampleTime=1
  cfblk2 : Outport
  cfblk15 : Outport  Port=2
  cfblk16 : Outport  Port=3
  wires:
  cfblk6/1 -> cfblk8/1
  cfblk11/1 -> cfblk16/1
  cfblk1/1 -> cfblk7/1
  cfblk9/1 -> cfblk4/1
  cfblk14/1 -> cfblk2/1
  cfblk10/1 -> cfblk3/1
  cfblk13/1 -> cfblk15/1
  cfblk7/1 -> cfblk5/1
  cfblk3/1 -> cfblk6/1

== system sampleModel1986/cfblk62 ==
  cfblk1 : Inport
  cfblk10 : Subsystem
  cfblk{12..15} (4 alike) : Delay  SampleTime=1
  cfblk3 : Squeeze
  cfblk4 : Reshape
  cfblk5 : Sum  Inputs=+-
  cfblk6 : Subsystem
  cfblk7 : Subsystem
  cfblk8 : Subsystem
  cfblk9 : Subsystem
  cfblk2 : Outport
  cfblk11 : Outport  Port=2
  wires:
  cfblk10/1(cfblk2) -> cfblk8/1(cfblk1)
  cfblk8/1(cfblk2) -> cfblk9/1(cfblk1)
  cfblk3/1 -> cfblk7/1(cfblk1)
  cfblk6/1(cfblk2) -> cfblk11/1
  cfblk6/2(cfblk10) -> cfblk2/1
  cfblk1/1 -> cfblk4/1, cfblk9/4(cfblk12), cfblk9/6(cfblk14)
  cfblk5/1 -> cfblk3/1
  cfblk4/1 -> cfblk5/1
  cfblk8/3(cfblk11) -> cfblk9/2(cfblk10), cfblk9/5(cfblk13)
  cfblk7/1(cfblk2) -> cfblk10/2(cfblk11)
  cfblk10/2(cfblk13) -> cfblk6/1(cfblk1)
  cfblk7/2(cfblk16) -> cfblk9/3(cfblk11)
  cfblk10/3(cfblk14) -> cfblk6/2(cfblk9)
  cfblk6/3(cfblk11) -> cfblk8/2(cfblk9)
  cfblk9/1(cfblk2) -> cfblk12/1
  cfblk12/1 -> cfblk10/3(cfblk12)
  cfblk9/2(cfblk15) -> cfblk13/1
  cfblk13/1 -> cfblk7/2(cfblk15)
  cfblk9/3(cfblk16) -> cfblk14/1
  cfblk14/1 -> cfblk5/2
  cfblk8/2(cfblk10) -> cfblk15/1
  cfblk15/1 -> cfblk10/1(cfblk1)

== system sampleModel1986/cfblk63 ==
  cfblk1 : Inport
  cfblk12 : Inport  Port=2
  cfblk13 : Inport  Port=3
  cfblk10 : Subsystem
  cfblk11 : Subsystem
  cfblk3 : DiscreteFilter  SampleTime=1
  cfblk4 : Delay  SampleTime=1
  cfblk5 : simulink/Discrete/Difference  ICPrevInput=0.0  OutMin=[]  OutMax=[]  OutDataTypeStr=Inherit: Inherit via back propagation  OutDataType=fixdt(1, 16)  OutScaling=2^-10  DoSatur=off
  cfblk6 : Delay  DelayLengthSource=Input port  SampleTime=1
      settings: InputPortMap=u0,p1
  cfblk7 : simulink/Discrete/Transfer Fcn Real Zero  ZeroZ=0.75  ICPrevInput=0.0  DoSatur=off
      settings: SourceProductBaseCode=SL
  cfblk8 : Trigonometry
  cfblk9 : Subsystem
  cfblk2 : Outport
  wires:
  cfblk4/1 -> cfblk8/1, cfblk9/5(cfblk11)
  cfblk6/1 -> cfblk3/1
  cfblk7/1 -> cfblk11/1(cfblk1), cfblk9/2(cfblk8)
  cfblk3/1 -> cfblk9/1(cfblk1)
  cfblk11/1(cfblk2) -> cfblk2/1
  cfblk10/1(cfblk2) -> cfblk6/1
  cfblk1/1 -> cfblk5/1
  cfblk13/1 -> cfblk7/1
  cfblk9/1(cfblk2) -> cfblk11/2(cfblk11)
  cfblk5/1 -> cfblk10/1(cfblk1)
  cfblk10/2(cfblk6) -> cfblk4/1
  cfblk8/1 -> cfblk6/2, cfblk9/3(cfblk9)
  cfblk10/3(cfblk7) -> cfblk11/3(cfblk12), cfblk9/4(cfblk10)
  cfblk12/1 -> cfblk11/4(cfblk13)

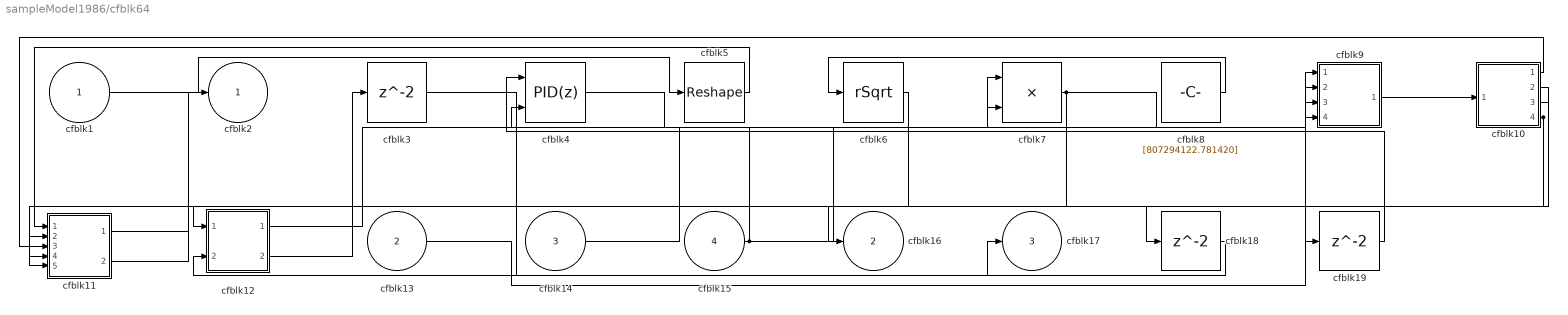
== system sampleModel1986/cfblk64 ==
  cfblk1 : Inport
  cfblk13 : Inport  Port=2
  cfblk14 : Inport  Port=3
  cfblk15 : Inport  Port=4
  cfblk10 : Subsystem
  cfblk11 : Subsystem
  cfblk12 : Subsystem
  cfblk18 : Delay  SampleTime=1
  cfblk19 : Delay  SampleTime=1
  cfblk3 : Delay  SampleTime=1
  cfblk4 : slpidlib/PID Controller (2DOF)  Controller=PID  Form=Parallel  TimeDomain=Discrete-time  UseExternalTs=off  SampleTime=1  IntegratorMethod=Forward Euler  FilterMethod=Forward Euler  ControllerParametersSource=internal  P=1  I=1  UseKiTs=off  D=0  N=100  UseFilter=on  b=1  c=1  TunerSelectOption=Transfer Function Based (PID Tuner App)  InitialConditionSource=internal  InitialConditionForIntegrator=0  InitialConditionForFilter=0  DifferentiatorICPrevScaledInput=0  ExternalReset=none  TrackingMode=off  Kt=1  LimitOutput=off  SatLimitsSource=internal  UpperSaturationLimit=inf  LowerSaturationLimit=-inf  LinearizeAsGain=off  AntiWindupMode=none  Kb=1  POutMin=[]  POutMax=[]  IOutMin=[]  IOutMax=[]  DOutMin=[]  DOutMax=[]  NOutMin=[]  NOutMax=[]  bOutMin=[]  bOutMax=[]  cOutMin=[]  cOutMax=[]  SumOutMin=[]  SumOutMax=[]  SaturationOutMin=[]  SaturationOutMax=[]  PParamMin=[]  PParamMax=[]  IParamMin=[]  IParamMax=[]  DParamMin=[]  DParamMax=[]  NParamMin=[]  NParamMax=[]  bParamMin=[]  bParamMax=[]  cParamMin=[]  cParamMax=[]  KbParamMin=[]  KbParamMax=[]  KtParamMin=[]  KtParamMax=[]  KbOutMin=[]  KbOutMax=[]  KtOutMin=[]  KtOutMax=[]  IntegratorOutMin=[]  IntegratorOutMax=[]  FilterOutMin=[]  FilterOutMax=[]  SumI1OutMin=[]  SumI1OutMax=[]  SumI2OutMin=[]  SumI2OutMax=[]  SumI3OutMin=[]  SumI3OutMax=[]  SumI4OutMin=[]  SumI4OutMax=[]  SumDOutMin=[]  SumDOutMax=[]  Sum1OutMin=[]  Sum1OutMax=[]  Sum2OutMin=[]  Sum2OutMax=[]  Sum3OutMin=[]  Sum3OutMax=[]  DifferentiatorOutMin=[]  DifferentiatorOutMax=[]  FilterDiffOutCoefMin=[]  FilterDiffOutCoefMax=[]  ReciprocalOutMin=[]  ReciprocalOutMax=[]  SumDenOutMin=[]  SumDenOutMax=[]  SumNumOutMin=[]  SumNumOutMax=[]  DivideOutMin=[]  DivideOutMax=[]  UdiffTsProdOutMin=[]  UdiffTsProdOutMax=[]  NTsProdOutMin=[]  NTsProdOutMax=[]  UintegralTsProdOutMin=[]  UintegralTsProdOutMax=[]  UngainTsProdOutMin=[]  UngainTsProdOutMax=[]  IntegratorContinuousStateAttributes=''  IntegratorStateMustResolveToSignalObject=off  IntegratorRTWStateStorageClass=Auto  FilterContinuousStateAttributes=''  FilterStateMustResolveToSignalObject=off  FilterRTWStateStorageClass=Auto  ParallelPVariant=InternalParameters  IdealPVariant=Disabled  IVariant=InternalParameters  DVariant=InternalParameters  bVariant=InternalParameters  cVariant=InternalParameters  IntegratorVariant=Discrete  SatVariant=Disabled  AWVariant=Passthrough  PCopyVariant=Disabled  TRVariant=Disabled  FdbkBlocksVariant=Forward  IdealPFdbkVariant=Disabled  SatFdbkVariant=Disabled  DerivativeFilterVariant=ForwardEulerFilter  NVariant=InternalParameters  NCopyVariant=Disabled  FilterICVariant=InternalICsFilter  IntegratorICVariant=InternalICs  ExternalResetVariant=Disabled  TRSumVariant=Passthrough  SumFdbkVariant=Disabled  SumVariant=Sum_PID  TsampFilterVariant=InternalTs  TsampNgainVariant=Passthrough  TsampIntegralVariant=Passthrough  ExternalSaturationOutDataTypeStr=Inherit: Same as second input
      settings: SourceProductBaseCode=SL
  cfblk5 : Reshape
  cfblk6 : Sqrt  Operator=rSqrt  AlgorithmType=Newton-Raphson
  cfblk7 : Product  Inputs=**
  cfblk8 : Constant  Value=[807294122.781420]  SampleTime=1
  cfblk9 : Subsystem
  cfblk2 : Outport
  cfblk16 : Outport  Port=2
  cfblk17 : Outport  Port=3
  wires:
  cfblk1/1 -> cfblk5/1
  cfblk8/1 -> cfblk6/1
  cfblk14/1 -> cfblk7/1
  cfblk3/1 -> cfblk17/1
  cfblk9/1(cfblk2) -> cfblk10/1(cfblk1)
  cfblk13/1 -> cfblk9/1(cfblk1)
  cfblk4/1 -> cfblk7/2
  cfblk15/1 -> cfblk9/2(cfblk10), cfblk4/2
  cfblk7/1 -> cfblk12/1(cfblk1), cfblk9/4(cfblk12)
  cfblk5/1 -> cfblk11/1(cfblk1)
  cfblk6/1 -> cfblk11/2(cfblk10)
  cfblk10/1(cfblk2) -> cfblk11/3(cfblk11)
  cfblk11/1(cfblk2) -> cfblk16/1
  cfblk12/1(cfblk2) -> cfblk9/3(cfblk11)
  cfblk11/2(cfblk14) -> cfblk2/1
  cfblk10/4(cfblk17) -> cfblk11/4(cfblk12), cfblk11/5(cfblk13)
  cfblk12/2(cfblk11) -> cfblk3/1
  cfblk10/2(cfblk15) -> cfblk18/1
  cfblk18/1 -> cfblk12/2(cfblk10)
  cfblk10/3(cfblk16) -> cfblk19/1
  cfblk19/1 -> cfblk4/1

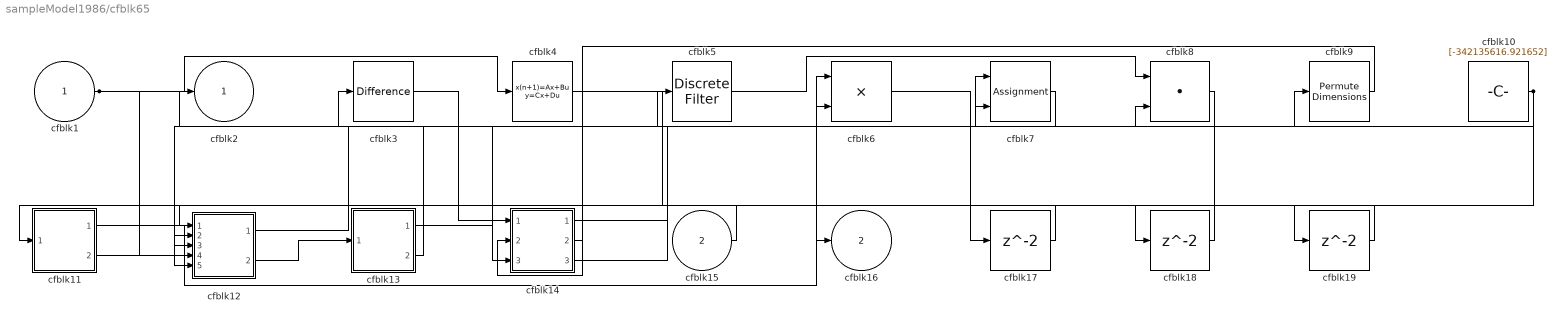
== system sampleModel1986/cfblk65 ==
  cfblk1 : Inport
  cfblk15 : Inport  Port=2
  cfblk10 : Constant  Value=[-342135616.921652]  SampleTime=1
  cfblk11 : Subsystem
  cfblk12 : Subsystem
  cfblk13 : Subsystem
  cfblk14 : Subsystem
  cfblk17 : Delay  SampleTime=1
  cfblk18 : Delay  SampleTime=1
  cfblk19 : Delay  SampleTime=1
  cfblk3 : simulink/Discrete/Difference  ICPrevInput=0.0  OutMin=[]  OutMax=[]  OutDataTypeStr=Inherit: Inherit via back propagation  OutDataType=fixdt(1, 16)  OutScaling=2^-10  DoSatur=off
  cfblk4 : DiscreteStateSpace
  cfblk5 : DiscreteFilter  SampleTime=1
  cfblk6 : Product
  cfblk7 : Assignment  DiagnosticForDimensions=Warning  IndexOptions=Index vector (dialog)  Indices=1  OutputSizes=1
  cfblk8 : DotProduct  OutDataTypeStr=Inherit: Inherit via internal rule
  cfblk9 : PermuteDimensions
  cfblk2 : Outport
  cfblk16 : Outport  Port=2
  wires:
  cfblk3/1 -> cfblk14/1(cfblk1)
  cfblk1/1 -> cfblk4/1, cfblk12/4(cfblk13)
  cfblk11/1(cfblk2) -> cfblk6/1
  cfblk5/1 -> cfblk8/1
  cfblk9/1 -> cfblk14/2(cfblk10)
  cfblk10/1 -> cfblk14/3(cfblk11), cfblk8/2, cfblk12/5(cfblk14)
  cfblk15/1 -> cfblk11/1(cfblk1)
  cfblk4/1 -> cfblk16/1
  cfblk7/1 -> cfblk6/2
  cfblk12/1(cfblk2) -> cfblk7/1
  cfblk14/2(cfblk12) -> cfblk2/1
  cfblk11/2(cfblk7) -> cfblk9/1
  cfblk12/2(cfblk15) -> cfblk13/1(cfblk1)
  cfblk14/3(cfblk13) -> cfblk7/2
  cfblk13/1(cfblk2) -> cfblk5/1
  cfblk13/2(cfblk8) -> cfblk3/1
  cfblk6/1 -> cfblk17/1
  cfblk17/1 -> cfblk12/3(cfblk12)
  cfblk8/1 -> cfblk18/1
  cfblk18/1 -> cfblk12/1(cfblk1)
  cfblk14/1(cfblk2) -> cfblk19/1
  cfblk19/1 -> cfblk12/2(cfblk11)
